simulink model "Part_E_AM_SSB_Modem"  (R2022b)
settings: Solver=VariableStepAuto  StartTime=0  StopTime=0.01  FixedStep=1/25000  RelTol=1e-3
values from neighbouring files (symbols this model uses):
  fs = 100000    [PART_D_SSB_USING_MATLAB.m]
libraries: commanapbnd3 x4
settings Model: Creator=dscmu  LastModifiedBy=dscmu

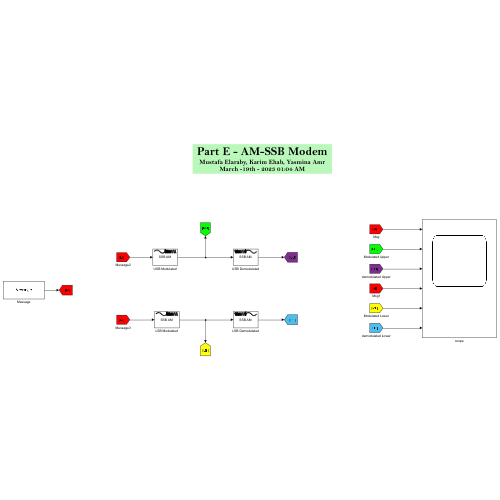
[thumbnail: Simulink's stored preview of the top-level diagram]
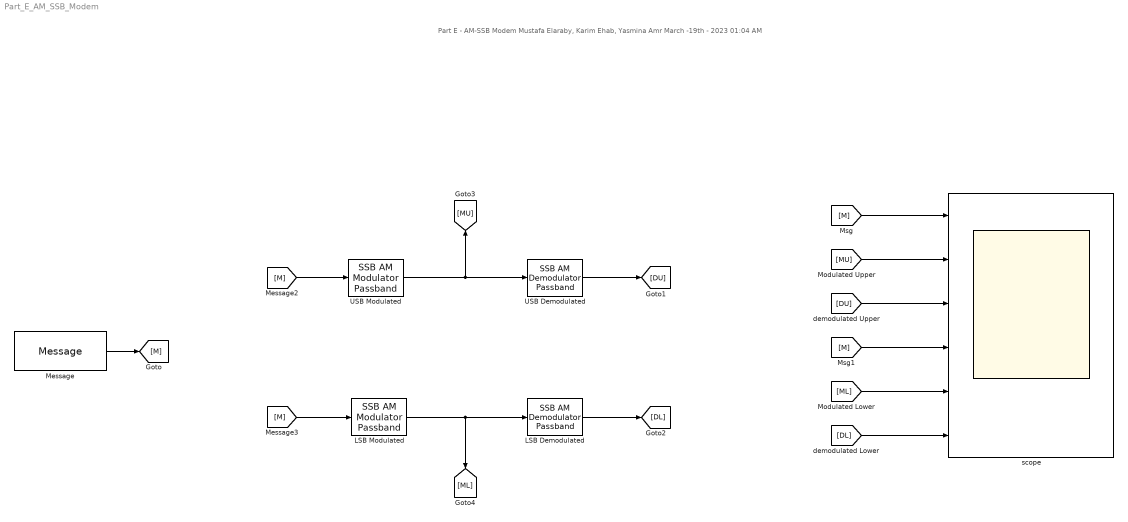
== system Part_E_AM_SSB_Modem ==
  note: Part E - AM-SSB Modem
      | Mustafa Elaraby, Karim Ehab, Yasmina Amr
      | March -19th - 2023 01:04 AM
  LSB Demodulated : commanapbnd3/SSB AM Demodulator Passband  Fc=10000  Ph=0  method=Butterworth  n=4  cf=2000  Rp=0.1  Rs=50
  LSB Modulated : commanapbnd3/SSB AM Modulator Passband  Fc=10000  Ph=0  Sd=Lower  Ho=4
  Message : FromWorkspace  VariableName=Message  SampleTime=1/fs
  USB Demodulated : commanapbnd3/SSB AM Demodulator Passband  Fc=10000  Ph=0  method=Butterworth  n=4  cf=2000  Rp=0.1  Rs=50
  USB Modulated : commanapbnd3/SSB AM Modulator Passband  Fc=10000  Ph=0  Sd=Upper  Ho=4
  scope : Scope  NumInputPorts=6
  wires:
  Message/1 -> [M]
  [M] -> scope/1
  USB Modulated/1 -> USB Demodulated/1, [MU]
  [MU] -> scope/2
  LSB Modulated/1 -> LSB Demodulated/1, [ML]
  [M] -> LSB Modulated/1
  [M] -> USB Modulated/1
  USB Demodulated/1 -> [DU]
  LSB Demodulated/1 -> [DL]
  [DU] -> scope/3
  [DL] -> scope/6
  [ML] -> scope/5
  [M] -> scope/4
